simulink model "simulacionrlc"  (R2020b)
settings: Solver=VariableStepAuto  StartTime=0.0  StopTime=0.7  MaxStep=1e-3  RelTol=1e-3
values from neighbouring files (symbols this model uses):
  C = 6e-6    (= 6e-06)    [sim_rlc.m]
  L = 1000e-3    (= 1)    [sim_rlc.m]
  R = 10e3    (= 10000)    [sim_rlc.m]
settings Model: Creator=Acer  LastModifiedBy=Acer

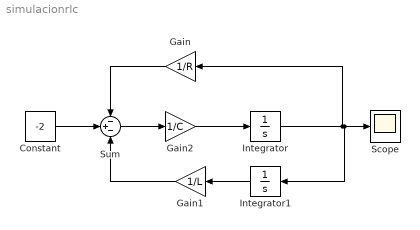
== system simulacionrlc ==
  Constant : Constant  Value=-2
  Gain : Gain  Gain=1/R
  Gain1 : Gain  Gain=1/L
  Gain2 : Gain  Gain=1/C
  Integrator : Integrator
  Integrator1 : Integrator
  Scope : Scope
  Sum : Sum  Inputs=-+-
  wires:
  Sum/1 -> Gain2/1
  Gain2/1 -> Integrator/1
  Integrator1/1 -> Gain1/1
  Gain1/1 -> Sum/3
  Integrator/1 -> Scope/1, Integrator1/1, Gain/1
  Gain/1 -> Sum/1
  Constant/1 -> Sum/2
